simulink model "Tip_SS"  (R2019b)
settings: Solver=FixedStepAuto  StartTime=0  StopTime=5  FixedStep=0.002  RelTol=1e-3  EnableMultiTasking=on
PostLoadFcn:
  | qc_set_target_type(getConfigSet(bdroot, 'QUARC Default Target Configuration'));
values from neighbouring files (symbols this model uses):
  L_obs = place(sysest_ct_tip.A',sysest_ct_tip.C', obs_poles)'    [main.m]
  sysest_ct = d2c(sysest)    [main.m]
  v_a_max = 13    [main.m]
undefined symbols (not defined in the file or in its folder): HIL, K_lqr_eta, K_lqr_x, K_p, K_pp, qc_get_step_size, sigbuilder_block
libraries: simulink_extras x7, quarc_library x4, cstblocks x1
settings Model: SimulationMode=external  ExtModeTrigDuration=5000  Creator=CFulford  LastModifiedBy=AleFire
settings SolverCC: PositivePriorityOrder=on
settings DataIOCC: LimitDataPoints=on  SaveFormat=Array  SignalLoggingSaveFormat=ModelDataLogs  ReturnWorkspaceOutputs=off
settings OptimizationCC: ExpressionDepthLimit=2147483647  InitFltsAndDblsToZero=on  LifeSpan=inf
settings DebuggingCC: SaveWithParameterizedLinksMsg=none  UnderspecifiedInitializationDetection=Classic  MergeDetectMultiDrivingBlocksExec=none  SolverPrmCheckMsg=warning  MultiTaskDSMMsg=warning  MultiTaskCondExecSysMsg=none  FcnCallInpInsideContextMsg=warning  StateNameClashWarn=warning  SFUnexpectedBacktrackingDiag=warning  SFNoUnconditionalDefaultTransitionDiag=warning  SFExecutionAtInitializationDiag=none  ArithmeticOperatorsInVariantConditions=warning
settings HardwareCC: ProdBitPerPointer=32  ProdBitPerSizeT=32  ProdBitPerPtrDiffT=32  ProdLargestAtomicFloat=None  ProdIntDivRoundTo=Undefined  ProdEndianess=Unspecified  ProdWordSize=32  ProdHWDeviceType=32-bit Generic
settings ModelReferenceCC: PropagateSignalLabelsOutOfModel=off
settings SFSimCC: SimUseLocalCustomCode=off  CustomCodeUndefinedFunction=UseInterfaceOnly
settings RTWCC: Description=QUARC Win64 Target  SystemTargetFile=quarc_win64.tlc  TemplateMakefile=quarc_default_tmf  RTWUseLocalCustomCode=off
settings CodeAppCC: StateflowObjectComments=on
settings STFCustomTargetCC: TargetPreCompLibLocation=C:\PROGRA~3\QUARC\lib\2019b\win64\release  ConcurrentExecutionCompliant=on  CombineOutputUpdateFcns=on  CPPClassGenCompliant=on  SystemTargetFile=quarc_win64.tlc
settings GRTTargetCC: TargetPreCompLibLocation=C:\PROGRA~3\QUARC\lib\2019b\win64\release  TargetLangStandard=C89/C90 (ANSI)  ParMdlRefBuildCompliant=off  CompOptLevelCompliant=off  MatFileLogging=off  UseToolchainInfoCompliant=off  ExtMode=on  ExtModeMexFile=quarc_comm
settings ConfigComp: CovMetricSettings=dw  CovSaveCumulativeToWorkspaceVar=on  CovSaveSingleToWorkspaceVar=on  CovExternalEMLEnable=off  CovSFcnEnable=off

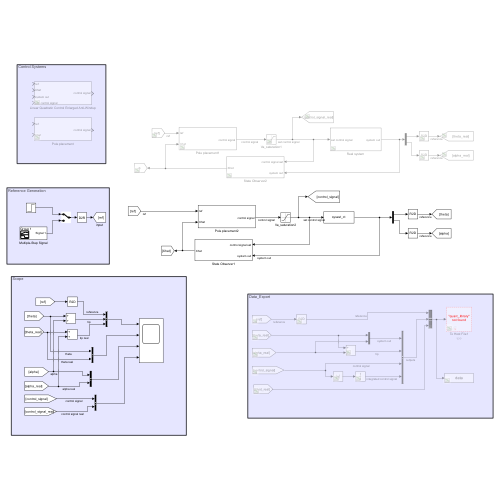
[thumbnail: Simulink's stored preview of the top-level diagram]
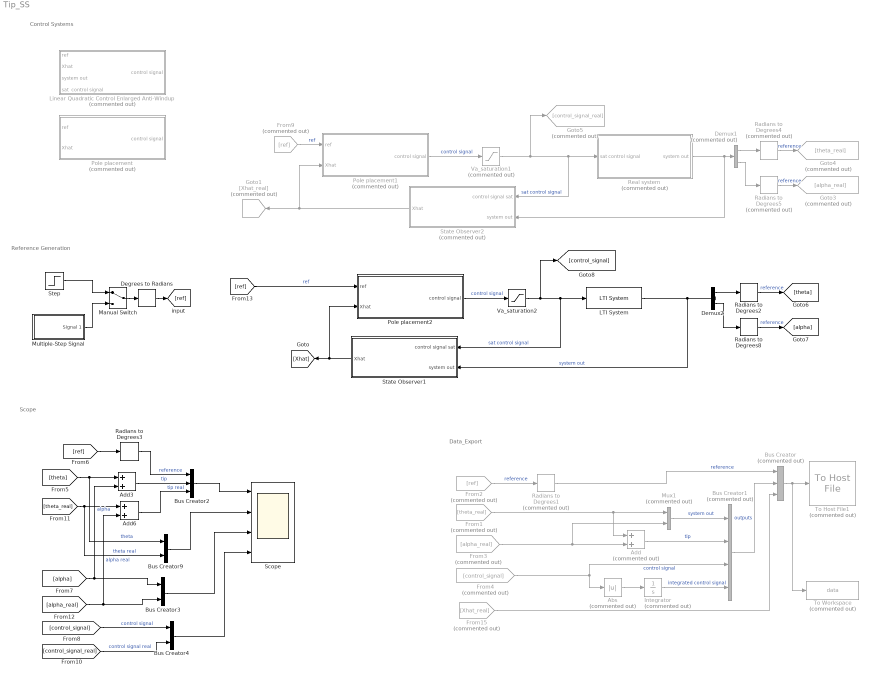
== system Tip_SS ==
  note: Control Systems
  note: Data_Export
  note: Reference Generation
  note: Scope
  Abs : Abs  Commented=on
  Add : Sum  Commented=on
  Add3 : Sum
  Add6 : Sum
  Bus Creator : BusCreator  Commented=on  Inputs=3
  Bus Creator1 : BusCreator  Commented=on  Inputs=4
  Bus Creator2 : BusCreator  Inputs=3
  Bus Creator3 : BusCreator  Inputs=2
  Bus Creator4 : BusCreator  Inputs=2
  Bus Creator9 : BusCreator  Inputs=2
  Degrees to Radians : simulink_extras/Transformations/Degrees to Radians
  Demux1 : Demux  Commented=on  Outputs=2
  Demux2 : Demux  Outputs=2
  From1 : From  Commented=on  GotoTag=theta_real
  From15 : From  Commented=on  GotoTag=Xhat_real
  From2 : From  Commented=on  GotoTag=ref
  From3 : From  Commented=on  GotoTag=alpha_real
  From4 : From  Commented=on  GotoTag=control_signal
  From9 : From  Commented=on  GotoTag=ref
  Goto1 : Goto  Commented=on  GotoTag=Xhat_real
  Goto3 : Goto  Commented=on  GotoTag=alpha_real
  Goto4 : Goto  Commented=on  GotoTag=theta_real
  Goto5 : Goto  Commented=on  GotoTag=control_signal_real
  Integrator : Integrator  Commented=on
  LTI System : cstblocks/LTI System  sys=sysest_ct  IC=[]
  Linear Quadratic Control Enlarged Anti-Windup : Subsystem  Commented=on
  Manual Switch : ManualSwitch
  Multiple-Step Signal : Subsystem  Tag=STV Subsys  LoadFcn=sigbuilder_block('load');  StartFcn=sigbuilder_block('start');  StopFcn=sigbuilder_block('stop');  ClipboardFcn=sigbuilder_block('clipboard');  mask(Sigbuilder block){tuvar=[0:10]}
      mask help: Simulink:masks:SigbuilderBlock_MD
      mask init:
      | if ~strcmp(get_param(bdroot(gcbh),'SimulationStatus'),'stopped') tuvar = sigbuilder_block('maskInit'); end
      settings: CopyFcn=sigbuilder_block('copy');  DeleteFcn=sigbuilder_block('delete');  ModelCloseFcn=sigbuilder_block('modelClose');  PreSaveFcn=sigbuilder_block('preSave');  PauseFcn=sigbuilder_block('pause');  ContinueFcn=sigbuilder_block('continue');  NameChangeFcn=sigbuilder_block('namechange');  OpenFcn=sigbuilder_block('open',[437.6 199.2 550.4 400 ]);  CloseFcn=sigbuilder_block('close');
      mask Display: plot(0, 0, 100, 100,[2, 2, 32, 32, 2], [68, 8, 8, 68, 68],[32, 2], [38, 38], [32, 19, 2],[53, 60, 44], [32, 17, 17, 2],[16, 16, 31, 31]);txt = getActiveGroup(gcbh);text(2, 100, txt,'verticalAlignment', 'top');
  Mux1 : Mux  Commented=on  Inputs=2
  Pole placement : Subsystem  Commented=on
  Pole placement1 : Subsystem  Commented=on
  Pole placement2 : Subsystem
  Radians to Degrees1 : simulink_extras/Transformations/Radians to Degrees  Commented=on
  Radians to Degrees2 : simulink_extras/Transformations/Radians to Degrees
  Radians to Degrees3 : simulink_extras/Transformations/Radians to Degrees
  Radians to Degrees4 : simulink_extras/Transformations/Radians to Degrees  Commented=on
  Radians to Degrees5 : simulink_extras/Transformations/Radians to Degrees  Commented=on
  Radians to Degrees8 : simulink_extras/Transformations/Radians to Degrees
  Real system : Subsystem  Commented=on
  Scope : Scope  NumInputPorts=4
  State Observer1 : Subsystem
  State Observer2 : Subsystem  Commented=on
  Step : Step  After=45  SampleTime=0
  To Host File1 : quarc_library/Sinks/To Host/To Host File  Commented=on  file_name=Sine tests\Sine_24_in_theta_alpha.mat  variable_name=data  decimation=1  sample_time=-1  file_format=MAT-file v.4  options=No header or footer  append=off  final_file_name=Sine tests\Sine_24_in_theta_alpha.mat  bitrate=2000000
  To Workspace : ToWorkspace  Commented=on  VariableName=data  SaveFormat=Timeseries  SampleTime=-1
  Va_saturation1 : Saturate  Commented=on  UpperLimit=v_a_max  LowerLimit=-v_a_max
  Va_saturation2 : Saturate  UpperLimit=v_a_max  LowerLimit=-v_a_max
  wires:
  Pole placement1/1(" control signal") -> Va_saturation1/1  "control signal"
  Demux2/1 -> Radians to Degrees2/1
  Pole placement2/1(" control signal") -> Va_saturation2/1  "control signal"
  [ref] -> Pole placement2/1(ref)  "ref"
  Demux1/1 -> Radians to Degrees4/1
  Va_saturation2/1 -> [control_signal], LTI System/1, State Observer1/1(control signal sat)  "sat control signal"
  Demux1/2 -> Radians to Degrees5/1
  LTI System/1 -> State Observer1/2(system out), Demux2/1  "system out"
  Va_saturation1/1 -> Goto5/1, State Observer2/1(control signal sat), Real system/1(sat control signal)  "sat control signal"
  Demux2/2 -> Radians to Degrees8/1
  From9/1 -> Pole placement1/1(ref)  "ref"
  Radians to Degrees2/1 -> [theta]  "reference"
  Radians to Degrees8/1 -> [alpha]  "reference"
  State Observer2/1(Xhat) -> Pole placement1/2(Xhat), Goto1/1
  Bus Creator/1 -> To Workspace/1, To Host File1/1
  From1/1 -> Add/1, Mux1/1
  From2/1 -> Radians to Degrees1/1  "reference"
  Abs/1 -> Integrator/1
  From4/1 -> Abs/1, Bus Creator1/3  "control signal"
  Mux1/1 -> Bus Creator1/1  "system out"
  Integrator/1 -> Bus Creator1/4  "integrated control signal"
  Radians to Degrees1/1 -> Bus Creator/1  "reference"
  Bus Creator1/1 -> Bus Creator/2  "outputs"
  From15/1 -> Bus Creator/3
  Add/1 -> Bus Creator1/2  "tip"
  From3/1 -> Add/2, Mux1/2
  Radians to Degrees4/1 -> Goto4/1  "reference"
  Radians to Degrees5/1 -> Goto3/1  "reference"
  State Observer1/1(Xhat) -> [Xhat], Pole placement2/2(Xhat)
  Real system/1(system out) -> State Observer2/2(system out), Demux1/1
  Multiple-Step Signal/1(Signal 1) -> Manual Switch/2
  Degrees to Radians/1 -> [ref]
  Manual Switch/1 -> Degrees to Radians/1
  Step/1 -> Manual Switch/1
  [ref] -> Radians to Degrees3/1
  Add6/1 -> Bus Creator2/3  "tip real"
  [control_signal] -> Bus Creator4/1  "control signal"
  Bus Creator2/1 -> Scope/1
  [control_signal_real] -> Bus Creator4/2  "control signal real"
  Add3/1 -> Bus Creator2/2  "tip"
  [alpha_real] -> Bus Creator3/2, Add6/2  "alpha real"
  [theta] -> Bus Creator9/1, Add3/1  "theta"
  Radians to Degrees3/1 -> Bus Creator2/1  "reference"
  Bus Creator4/1 -> Scope/4
  Bus Creator3/1 -> Scope/3
  Bus Creator9/1 -> Scope/2
  [theta_real] -> Bus Creator9/2, Add6/1  "theta real"
  [alpha] -> Bus Creator3/1, Add3/2  "alpha"

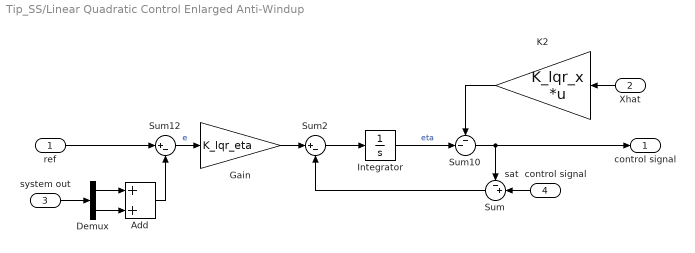
== system Tip_SS/Linear Quadratic Control Enlarged Anti-Windup ==
  ref : Inport
  Xhat : Inport  Port=2
  system out : Inport  Port=3
  sat  control signal : Inport  Port=4
  Add : Sum
  Demux : Demux  Outputs=2
  Gain : Gain  Gain=K_lqr_eta
  Integrator : Integrator
  K2 : Gain  Gain=K_lqr_x  Multiplication=Matrix(K*u)
  Sum : Sum  Inputs=-+|
  Sum10 : Sum  Inputs=--|
  Sum12 : Sum  Inputs=|+-
  Sum2 : Sum  Inputs=|+-
  " control signal" : Outport
  wires:
  ref/1 -> Sum12/1
  Integrator/1 -> Sum10/2  "eta"
  K2/1 -> Sum10/1
  Add/1 -> Sum12/2
  Xhat/1 -> K2/1
  system out/1 -> Demux/1
  Demux/2 -> Add/2
  Demux/1 -> Add/1
  sat  control signal/1 -> Sum/2
  Sum10/1 -> " control signal"/1, Sum/1
  Sum12/1 -> Gain/1  "e"
  Sum2/1 -> Integrator/1
  Sum/1 -> Sum2/2
  Gain/1 -> Sum2/1

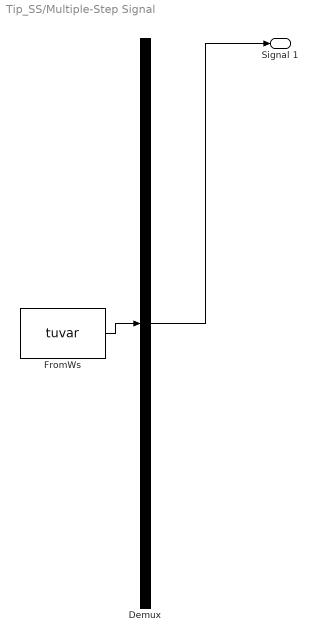
== system Tip_SS/Multiple-Step Signal ==
  Demux : Demux  Tag=STV Demux  Outputs=1
      settings: DisplayOption=none
  FromWs : FromWorkspace  Tag=STV FromWs  VariableName=tuvar
      SigBuilderData=|
      | common.afterFinalStr = 'Extrapolate'
      | common.sampleTime = 0
      | dataSet.timeRange = [0 10]
      | dataSet.name = 'Group 1'
      | sbobj.Groups.Name = 'Group 1'
      | sbobj.Groups.Signals.Name = 'Signal 1'
      | sbobj.Groups.Signals.XData = [0 1 1 3 3 5 5 7 7 8.5 8.5 10]
      | sbobj.Groups.Signals.YData = [0.005 0.005 40 40 15 15 -30 -30 0 0 23 23]
  Signal 1 : Outport  Tag=STV Outport
  wires:
  Demux/1 -> Signal 1/1
  FromWs/1 -> Demux/1

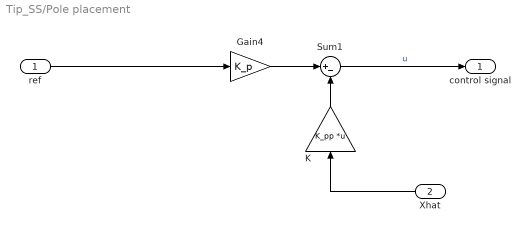
== system Tip_SS/Pole placement ==
  ref : Inport
  Xhat : Inport  Port=2
  Gain4 : Gain  Gain=K_p
  K : Gain  Gain=K_pp  Multiplication=Matrix(K*u)
  Sum1 : Sum  Inputs=|+-
  " control signal" : Outport
  wires:
  K/1 -> Sum1/2
  Xhat/1 -> K/1
  Sum1/1 -> " control signal"/1  "u"
  Gain4/1 -> Sum1/1
  ref/1 -> Gain4/1

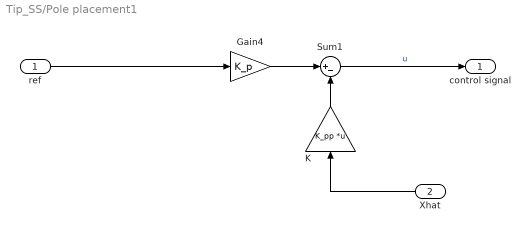
== system Tip_SS/Pole placement1 ==
  ref : Inport
  Xhat : Inport  Port=2
  Gain4 : Gain  Gain=K_p
  K : Gain  Gain=K_pp  Multiplication=Matrix(K*u)
  Sum1 : Sum  Inputs=|+-
  " control signal" : Outport
  wires:
  K/1 -> Sum1/2
  Xhat/1 -> K/1
  Sum1/1 -> " control signal"/1  "u"
  Gain4/1 -> Sum1/1
  ref/1 -> Gain4/1

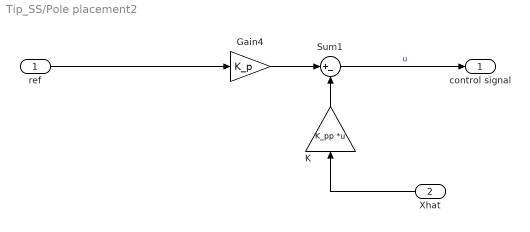
== system Tip_SS/Pole placement2 ==
  ref : Inport
  Xhat : Inport  Port=2
  Gain4 : Gain  Gain=K_p
  K : Gain  Gain=K_pp  Multiplication=Matrix(K*u)
  Sum1 : Sum  Inputs=|+-
  " control signal" : Outport
  wires:
  K/1 -> Sum1/2
  Xhat/1 -> K/1
  Sum1/1 -> " control signal"/1  "u"
  Gain4/1 -> Sum1/1
  ref/1 -> Gain4/1

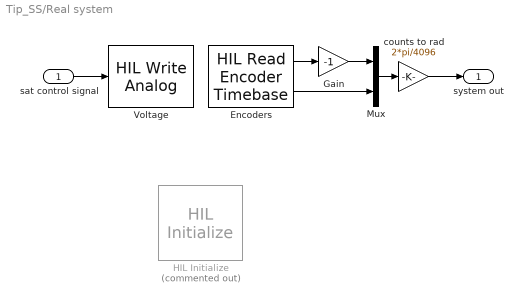
== system Tip_SS/Real system ==
  sat control signal : Inport
  Encoders : quarc_library/Data Acquisition/Generic/Timebases/HIL Read Encoder Timebase  object_name=HIL-1  clock=0  channels=[0:1]  samples_in_buffer=max(ceil(1/qc_get_step_size), 1)  active=on  vector_output=off  data_type_mode=Inherit via back propagation  data_type=double
  Gain : Gain  Gain=-1
  HIL Initialize : quarc_library/Data Acquisition/Generic/Configuration/HIL Initialize  Priority=-99  Commented=on  object_name=HIL-1  board_type=q2_usb  board_number=0  board_options=d0=digital;d1=digital;led=auto;update_rate=normal;decimation=1  exclusive=off  active=off  hardware_clocks=[0]  clock_modes=[]  initial_clock_frequencies=[]  set_clock_params_at_start=off  set_clock_params_at_switch_in=off  set_clock_frequencies_at_start=off  set_clock_frequencies_at_switch_in=off  analog_input_channels=[0:1]  analog_input_configurations=[]  analog_input_maximums=10  analog_input_minimums=-10  set_analog_input_params_at_start=on  set_analog_input_params_at_switch_in=off  analog_output_channels=[0:1]  analog_output_maximums=10  analog_output_minimums=-10  initial_analog_outputs=[0]  final_analog_outputs=[0]  watchdog_analog_outputs=0  set_analog_output_params_at_start=on  set_analog_output_params_at_switch_in=off  set_analog_outputs_at_start=on  set_analog_outputs_at_switch_in=off  set_analog_outputs_at_terminate=on  set_analog_outputs_at_switch_out=off  set_analog_outputs_on_watchdog=off  digital_input_channels=[]  digital_output_channels=[]  digital_output_configuration=[]  initial_digital_outputs=[1]  final_digital_outputs=[1]  watchdog_digital_outputs=[1]  set_digital_output_params_at_start=off  set_digital_output_params_at_switch_in=off  set_digital_outputs_at_start=on  set_digital_outputs_at_switch_in=off  set_digital_outputs_at_terminate=on  set_digital_outputs_at_switch_out=off  set_digital_outputs_on_watchdog=off  encoder_channels=[0:1]  quadrature=[4]  encoder_filter_frequency=[]  initial_encoder_counts=[0]  set_encoder_params_at_start=on  set_encoder_params_at_switch_in=off  set_encoder_counts_at_start=on  set_encoder_counts_at_switch_in=off  pwm_channels=[]  pwm_modes=[0]  pwm_frequency=1/0.020  pwm_configuration=[]  pwm_alignment=[]  pwm_polarity=[]  pwm_leading_deadband=[]  pwm_trailing_deadband=[]  initial_pwm_outputs=[0]  final_pwm_outputs=[0]  watchdog_pwm_outputs=[0]  set_pwm_params_at_start=on  set_pwm_params_at_switch_in=off  set_pwm_outputs_at_start=on  set_pwm_outputs_at_switch_in=off  set_pwm_outputs_at_terminate=on  set_pwm_outputs_at_switch_out=off  set_pwm_outputs_on_watchdog=off  other_output_channels=[]  initial_other_outputs=[]  final_other_outputs=[]  watchdog_other_outputs=[]  set_other_outputs_at_start=off  set_other_outputs_at_switch_in=off  set_other_outputs_at_terminate=off  set_other_outputs_at_switch_out=off  set_other_outputs_on_watchdog=off
  Mux : Mux  Inputs=2
  Voltage : quarc_library/Data Acquisition/Generic/Immediate I//O/HIL Write Analog  object_name=HIL-1  channels=0  sample_time=-1  active=off  vector_input=off
  counts to rad : Gain  Gain=2*pi/4096
  system out : Outport
  wires:
  sat control signal/1 -> Voltage/1
  Encoders/1 -> Gain/1
  Encoders/2 -> Mux/2
  Mux/1 -> counts to rad/1
  Gain/1 -> Mux/1
  counts to rad/1 -> system out/1

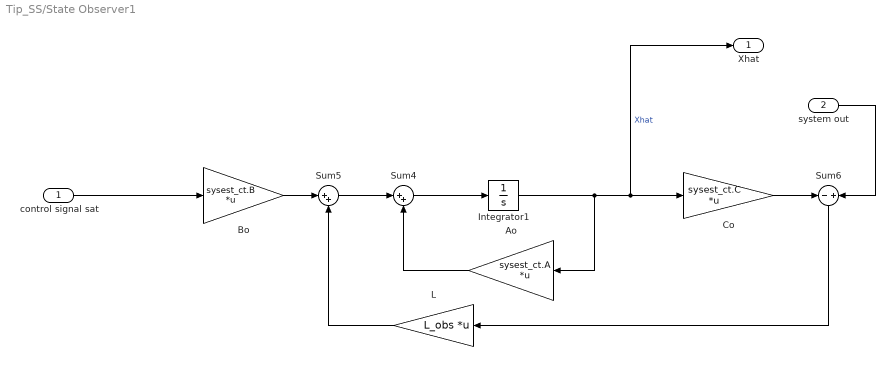
== system Tip_SS/State Observer1 ==
  control signal sat : Inport
  system out : Inport  Port=2
  Ao : Gain  Gain=sysest_ct.A  Multiplication=Matrix(K*u)
  Bo : Gain  Gain=sysest_ct.B  Multiplication=Matrix(K*u)
  Co : Gain  Gain=sysest_ct.C  Multiplication=Matrix(K*u)
  Integrator1 : Integrator
  L : Gain  Gain=L_obs  Multiplication=Matrix(K*u)
  Sum4 : Sum  Inputs=|++
  Sum5 : Sum  Inputs=|++
  Sum6 : Sum  Inputs=-+
  Xhat : Outport
  wires:
  system out/1 -> Sum6/2
  Ao/1 -> Sum4/2
  Sum4/1 -> Integrator1/1
  control signal sat/1 -> Bo/1
  Co/1 -> Sum6/1
  Sum6/1 -> L/1
  Bo/1 -> Sum5/1
  L/1 -> Sum5/2
  Integrator1/1 -> Xhat/1, Co/1, Ao/1  "Xhat"
  Sum5/1 -> Sum4/1

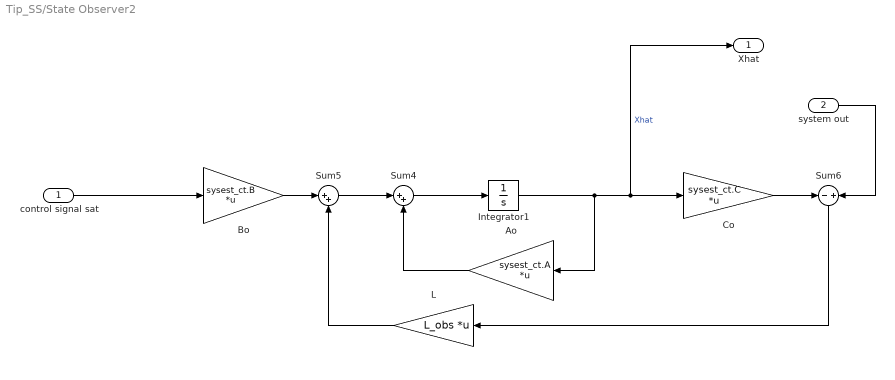
== system Tip_SS/State Observer2 ==
  control signal sat : Inport
  system out : Inport  Port=2
  Ao : Gain  Gain=sysest_ct.A  Multiplication=Matrix(K*u)
  Bo : Gain  Gain=sysest_ct.B  Multiplication=Matrix(K*u)
  Co : Gain  Gain=sysest_ct.C  Multiplication=Matrix(K*u)
  Integrator1 : Integrator
  L : Gain  Gain=L_obs  Multiplication=Matrix(K*u)
  Sum4 : Sum  Inputs=|++
  Sum5 : Sum  Inputs=|++
  Sum6 : Sum  Inputs=-+
  Xhat : Outport
  wires:
  system out/1 -> Sum6/2
  Ao/1 -> Sum4/2
  Sum4/1 -> Integrator1/1
  control signal sat/1 -> Bo/1
  Co/1 -> Sum6/1
  Sum6/1 -> L/1
  Bo/1 -> Sum5/1
  L/1 -> Sum5/2
  Integrator1/1 -> Xhat/1, Co/1, Ao/1  "Xhat"
  Sum5/1 -> Sum4/1
